simulink model "HANcoder_E407_GTSync_v4"  (R2018b)
settings: Solver=FixedStepDiscrete  StartTime=0.0  StopTime=1  FixedStep=0.01  RelTol=1e-3
PreLoadFcn:
  | librarySetup
  | eval([bdroot,'_startup']) %Calling [modelName]_startup.m
values from neighbouring files (symbols this model uses):
  basic_cycle_duration = TM12 + COMP_duration    (= 495)    [HANcoder_E407_GTSync_v4_startup.m]
  COM_Period = 100    [HANcoder_E407_GTSync_v4_startup.m]
  COM_Phase = COM_Period/2    (= 50)    [HANcoder_E407_GTSync_v4_startup.m]
  comm_delay_estimation = 20    [HANcoder_E407_GTSync_v4_startup.m]
  frequency_IRQ = 20    [HANcoder_E407_GTSync_v4_startup.m]
  HANtuneOverride = Simulink.Parameter    [HANcoder_E407_GTSync_v4_startup.m]
  idle_time_init = basic_cycle_duration*matrix_rows    (= 990)    [HANcoder_E407_GTSync_v4_startup.m]
  LED_ticks_toggle = 10000    [HANcoder_E407_GTSync_v4_startup.m]
  Master_Role = 1    [HANcoder_E407_GTSync_v4_startup.m]
  matrix_rows = 2    [HANcoder_E407_GTSync_v4_startup.m]
  Slave_Role = 2    [HANcoder_E407_GTSync_v4_startup.m]
  Sync_ID = 1    [HANcoder_E407_GTSync_v4_startup.m]
  time_difference_threshold = 500    [HANcoder_E407_GTSync_v4_startup.m]
  TM0 = basic_cycle_start    (= 5)    [HANcoder_E407_GTSync_v4_startup.m]
  TM1 = TM0 + COMM_duration    (= 105)    [HANcoder_E407_GTSync_v4_startup.m]
  TM10 = TM9  + COMP_duration    (= 465)    [HANcoder_E407_GTSync_v4_startup.m]
  TM11 = TM10 + COMP_duration    (= 475)    [HANcoder_E407_GTSync_v4_startup.m]
  TM12 = TM11 + COMP_duration    (= 485)    [HANcoder_E407_GTSync_v4_startup.m]
  TM2 = TM1 + COMP_duration    (= 115)    [HANcoder_E407_GTSync_v4_startup.m]
  TM3 = TM2 + COMP_duration    (= 125)    [HANcoder_E407_GTSync_v4_startup.m]
  TM4 = TM3 + COMM_duration    (= 225)    [HANcoder_E407_GTSync_v4_startup.m]
  TM5 = TM4 + COMP_duration    (= 235)    [HANcoder_E407_GTSync_v4_startup.m]
  TM6 = TM5 + COMM_duration    (= 335)    [HANcoder_E407_GTSync_v4_startup.m]
  TM7 = TM6 + COMP_duration    (= 345)    [HANcoder_E407_GTSync_v4_startup.m]
  TM8 = TM7 + COMM_duration    (= 445)    [HANcoder_E407_GTSync_v4_startup.m]
  TM9 = TM8  + COMP_duration    (= 455)    [HANcoder_E407_GTSync_v4_startup.m]
  Vote1_ID = 12    [HANcoder_E407_GTSync_v4_startup.m]
  Vote2_ID = 22    [HANcoder_E407_GTSync_v4_startup.m]
  Vote3_ID = 32    [HANcoder_E407_GTSync_v4_startup.m]
  wrap_up_threshold = basic_cycle_duration - time_difference_threshold*10    (= -4505)    [HANcoder_E407_GTSync_v4_startup.m]
undefined symbols (not defined in the file or in its folder): A0, A1, CON2
libraries: HANcoder_STM32_Target x22, simulink x3, hdlsllib x2, simulink_extras x1
(part 2 of 5)

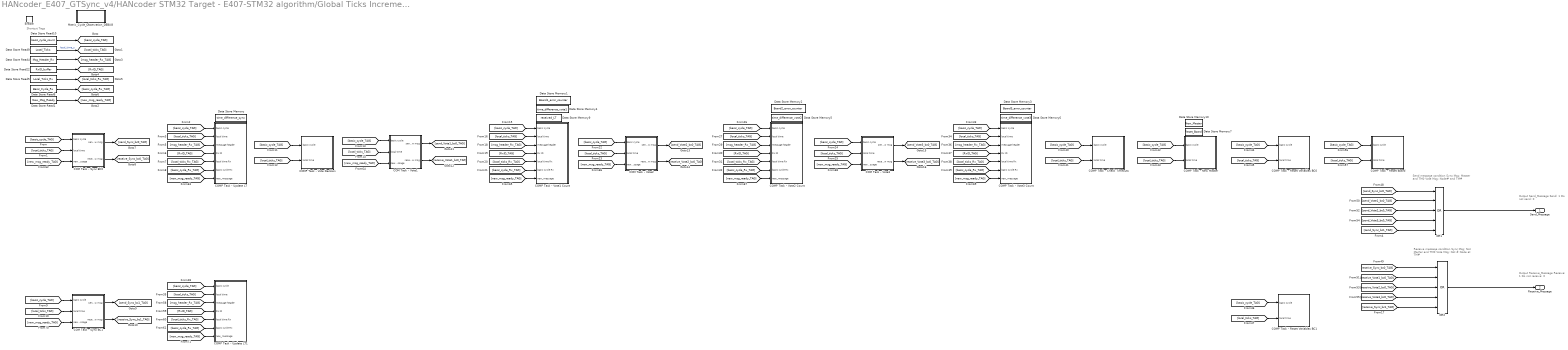
== system HANcoder_E407_GTSync_v4/HANcoder STM32 Target - E407-STM32 algorithm/Global Ticks Increment/CAN Management/Matrix Cycle Manager ==
  note: Receive message condition
      | Sync Msg: Not Master and TM0
      | Vote Msg: Not # Node at TM#
  note: Shortcut Tags
  note: Output Send_Message
      | Send: 1
      | Do not send: 0
  note: Send message condition
      | Sync Msg: Master and TM0
      | Vote Msg: Node# and TM#
  note: Output Receive_Message
      | Receive: 1
      | Do not receive: 0
  Enable : EnablePort  PropagateVarSize=During execution
  COM Task - Sync BC0 : Subsystem
  COM Task - Sync BC1 : Subsystem
  COM Task - Vote1 : Subsystem
  COM Task - Vote2 : Subsystem
  COM Task - Vote3 : Subsystem
  COMP Task - Check Timeouts : Subsystem
  COMP Task - New Master : Subsystem
  COMP Task - Reset Board : Subsystem
  COMP Task - Reset Variables BC0 : Subsystem
  COMP Task - Reset Variables BC1 : Subsystem
  COMP Task - Update LT : Subsystem
  COMP Task - Update LT1 : Subsystem
  COMP Task - Vote Decision : Subsystem
  COMP Task - Vote1 Count : Subsystem
  COMP Task - Vote2 Count : Subsystem
  COMP Task - Vote3 Count : Subsystem
  Data Store Memory : DataStoreMemory  DataStoreName=time_difference_sync  ReadBeforeWriteMsg=warning  WriteAfterWriteMsg=warning  WriteAfterReadMsg=warning  ShowAdditionalParam=off
  Data Store Memory1 : DataStoreMemory  DataStoreName=Board1_error_counter  ReadBeforeWriteMsg=warning  WriteAfterWriteMsg=warning  WriteAfterReadMsg=warning  ShowAdditionalParam=off  OutMin=0  OutMax=4294967294  OutDataTypeStr=double
  Data Store Memory10 : DataStoreMemory  DataStoreName=New_Master  ReadBeforeWriteMsg=warning  WriteAfterWriteMsg=warning  WriteAfterReadMsg=warning  ShowAdditionalParam=off  OutDataTypeStr=boolean
  Data Store Memory2 : DataStoreMemory  DataStoreName=Board2_error_counter  ReadBeforeWriteMsg=warning  WriteAfterWriteMsg=warning  WriteAfterReadMsg=warning  ShowAdditionalParam=off  OutMin=0  OutMax=4294967294  OutDataTypeStr=double
  Data Store Memory3 : DataStoreMemory  DataStoreName=Board3_error_counter  ReadBeforeWriteMsg=warning  WriteAfterWriteMsg=warning  WriteAfterReadMsg=warning  ShowAdditionalParam=off  OutMin=0  OutMax=4294967294  OutDataTypeStr=double
  Data Store Memory4 : DataStoreMemory  DataStoreName=time_difference_vote1  ReadBeforeWriteMsg=warning  WriteAfterWriteMsg=warning  WriteAfterReadMsg=warning  ShowAdditionalParam=off
  Data Store Memory5 : DataStoreMemory  DataStoreName=time_difference_vote2  ReadBeforeWriteMsg=warning  WriteAfterWriteMsg=warning  WriteAfterReadMsg=warning  ShowAdditionalParam=off
  Data Store Memory6 : DataStoreMemory  DataStoreName=time_difference_vote3  ReadBeforeWriteMsg=warning  WriteAfterWriteMsg=warning  WriteAfterReadMsg=warning  ShowAdditionalParam=off
  Data Store Memory7 : DataStoreMemory  DataStoreName=Reset_Board  ReadBeforeWriteMsg=warning  WriteAfterWriteMsg=warning  WriteAfterReadMsg=warning  ShowAdditionalParam=off  OutDataTypeStr=boolean
  Data Store Memory9 : DataStoreMemory  DataStoreName=received_LT  ReadBeforeWriteMsg=warning  WriteAfterWriteMsg=warning  WriteAfterReadMsg=warning  ShowAdditionalParam=off  OutDataTypeStr=Bus: received_vote_local_time
  Data Store Read1 : DataStoreRead  DataStoreName=New_Msg_Ready
  Data Store Read10 : DataStoreRead  DataStoreName=basic_cycle_count
  Data Store Read22 : DataStoreRead  DataStoreName=RxID_buffer
  Data Store Read4 : DataStoreRead  DataStoreName=Msg_Header_Rx
  Data Store Read5 : DataStoreRead  DataStoreName=Local_Ticks_Rx
  Data Store Read6 : DataStoreRead  DataStoreName=Basic_Cycle_Rx
  Data Store Read9 : DataStoreRead  DataStoreName=Local_Ticks
  Matrix_Cycle_Observation_DEBUG : Subsystem
  OR1 : Logic  Operator=OR  Inputs=5  IconShape=distinctive  AllPortsSameDT=off  OutDataTypeStr=boolean
  OR2 : Logic  Operator=OR  Inputs=5  IconShape=distinctive  AllPortsSameDT=off  OutDataTypeStr=boolean
  Send_Message : Outport
  Receive_Message : Outport  Port=2
  wires:
  Data Store Read10/1 -> [basic_cycle_TAG]
  OR1/1 -> Send_Message/1
  Data Store Read9/1 -> [local_ticks_TAG]  "local_time_s"
  Data Store Read4/1 -> [msg_header_Rx_TAG]
  Data Store Read22/1 -> [RxID_TAG]
  Data Store Read5/1 -> [local_ticks_Rx_TAG]
  Data Store Read6/1 -> [basic_cycle_Rx_TAG]
  [basic_cycle_TAG] -> COM Task - Sync BC0/1(basic cycle)
  [local_ticks_TAG] -> COM Task - Sync BC0/2(local time)
  [basic_cycle_TAG] -> COMP Task - Update LT/1(basic cycle)
  [local_ticks_TAG] -> COMP Task - Update LT/2(local time)
  COM Task - Sync BC0/1(send new msg) -> [send_Sync_bc0_TAG]
  COM Task - Sync BC0/2(receive new msg) -> [receive_Sync_bc0_TAG]
  [msg_header_Rx_TAG] -> COMP Task - Update LT/3(message header)
  [RxID_TAG] -> COMP Task - Update LT/4(Rx ID)
  [local_ticks_Rx_TAG] -> COMP Task - Update LT/5(local time Rx)
  [basic_cycle_Rx_TAG] -> COMP Task - Update LT/6(basic cycle Rx)
  COM Task - Sync BC1/2(receive new msg) -> [receive_Sync_bc1_TAG]
  COM Task - Sync BC1/1(send new msg) -> [send_Sync_bc1_TAG]
  [local_ticks_TAG] -> COM Task - Sync BC1/2(local time)
  [basic_cycle_TAG] -> COM Task - Sync BC1/1(basic cycle)
  [local_ticks_TAG] -> COMP Task - Vote Decision/2(local time)
  [basic_cycle_TAG] -> COMP Task - Vote Decision/1(basic cycle)
  COM Task - Vote1/2(receive new msg) -> [receive_Vote1_bc0_TAG]
  COM Task - Vote1/1(send new msg) -> [send_Vote1_bc0_TAG]
  [local_ticks_TAG] -> COM Task - Vote1/2(local time)
  [basic_cycle_TAG] -> COM Task - Vote1/1(basic cycle)
  [basic_cycle_Rx_TAG] -> COMP Task - Vote1 Count/6(basic cycle Rx)
  [local_ticks_Rx_TAG] -> COMP Task - Vote1 Count/5(local time Rx)
  [RxID_TAG] -> COMP Task - Vote1 Count/4(Rx ID)
  [msg_header_Rx_TAG] -> COMP Task - Vote1 Count/3(message header)
  [local_ticks_TAG] -> COMP Task - Vote1 Count/2(local time)
  [basic_cycle_TAG] -> COMP Task - Vote1 Count/1(basic cycle)
  [basic_cycle_TAG] -> COM Task - Vote2/1(basic cycle)
  [local_ticks_TAG] -> COM Task - Vote2/2(local time)
  COM Task - Vote2/1(send new msg) -> [send_Vote2_bc0_TAG]
  COM Task - Vote2/2(receive new msg) -> [receive_Vote2_bc0_TAG]
  COM Task - Vote3/2(receive new msg) -> [receive_Vote3_bc0_TAG]
  COM Task - Vote3/1(send new msg) -> [send_Vote3_bc0_TAG]
  [local_ticks_TAG] -> COM Task - Vote3/2(local time)
  [basic_cycle_TAG] -> COM Task - Vote3/1(basic cycle)
  [basic_cycle_TAG] -> COMP Task - Vote2 Count/1(basic cycle)
  [local_ticks_TAG] -> COMP Task - Vote2 Count/2(local time)
  [msg_header_Rx_TAG] -> COMP Task - Vote2 Count/3(message header)
  [RxID_TAG] -> COMP Task - Vote2 Count/4(Rx ID)
  [local_ticks_Rx_TAG] -> COMP Task - Vote2 Count/5(local time Rx)
  [basic_cycle_Rx_TAG] -> COMP Task - Vote2 Count/6(basic cycle Rx)
  [basic_cycle_Rx_TAG] -> COMP Task - Vote3 Count/6(basic cycle Rx)
  [local_ticks_Rx_TAG] -> COMP Task - Vote3 Count/5(local time Rx)
  [RxID_TAG] -> COMP Task - Vote3 Count/4(Rx ID)
  [msg_header_Rx_TAG] -> COMP Task - Vote3 Count/3(message header)
  [local_ticks_TAG] -> COMP Task - Vote3 Count/2(local time)
  [basic_cycle_TAG] -> COMP Task - Vote3 Count/1(basic cycle)
  [basic_cycle_TAG] -> COMP Task - Check Timeouts/1(basic cycle)
  [local_ticks_TAG] -> COMP Task - Check Timeouts/2(local time)
  [local_ticks_TAG] -> COMP Task - New Master/2(local time)
  [basic_cycle_TAG] -> COMP Task - New Master/1(basic cycle)
  [basic_cycle_TAG] -> COMP Task - Reset Variables BC0/1(basic cycle)
  [local_ticks_TAG] -> COMP Task - Reset Variables BC0/2(local time)
  [local_ticks_TAG] -> COMP Task - Reset Variables BC1/2(local time)
  [basic_cycle_TAG] -> COMP Task - Reset Variables BC1/1(basic cycle)
  [send_Sync_bc0_TAG] -> OR1/1
  [send_Vote1_bc0_TAG] -> OR1/2
  [send_Vote2_bc0_TAG] -> OR1/3
  [send_Vote3_bc0_TAG] -> OR1/4
  [receive_Vote3_bc0_TAG] -> OR2/4
  [receive_Vote2_bc0_TAG] -> OR2/3
  [receive_Vote1_bc0_TAG] -> OR2/2
  [receive_Sync_bc0_TAG] -> OR2/1
  [local_ticks_TAG] -> COMP Task - Reset Board/2(local time)
  [basic_cycle_TAG] -> COMP Task - Reset Board/1(basic cycle)
  OR2/1 -> Receive_Message/1
  [send_Sync_bc1_TAG] -> OR1/5
  [receive_Sync_bc1_TAG] -> OR2/5
  [basic_cycle_Rx_TAG] -> COMP Task - Update LT1/6(basic cycle Rx)
  [local_ticks_Rx_TAG] -> COMP Task - Update LT1/5(local time Rx)
  [RxID_TAG] -> COMP Task - Update LT1/4(Rx ID)
  [msg_header_Rx_TAG] -> COMP Task - Update LT1/3(message header)
  [local_ticks_TAG] -> COMP Task - Update LT1/2(local time)
  [basic_cycle_TAG] -> COMP Task - Update LT1/1(basic cycle)
  Data Store Read1/1 -> [new_msg_ready_TAG]
  [new_msg_ready_TAG] -> COM Task - Sync BC0/3(new_message)
  [new_msg_ready_TAG] -> COMP Task - Update LT/7(new_message)
  [new_msg_ready_TAG] -> COM Task - Vote1/3(new_message)
  [new_msg_ready_TAG] -> COMP Task - Vote1 Count/7(new_message)
  [new_msg_ready_TAG] -> COM Task - Vote2/3(new_message)
  [new_msg_ready_TAG] -> COMP Task - Vote2 Count/7(new_message)
  [new_msg_ready_TAG] -> COM Task - Vote3/3(new_message)
  [new_msg_ready_TAG] -> COMP Task - Vote3 Count/7(new_message)
  [new_msg_ready_TAG] -> COM Task - Sync BC1/3(new_message)
  [new_msg_ready_TAG] -> COMP Task - Update LT1/7(new_message)

== system HANcoder_E407_GTSync_v4/HANcoder STM32 Target - E407-STM32 algorithm/Global Ticks Increment/CAN Recieve/Buffer ready ==
  note: CAN_Rx - Buffer
      | ready for new message
  note: Logic Analyzer - DEBUG
      | Rx Buffer Ready
  Enable : EnablePort
  Data Store Write : DataStoreWrite  DataStoreName=Rx_State
  Data Store Write1 : DataStoreWrite  DataStoreName=Toggle_Pin
  New_Msg : Constant  Value=2  OutDataTypeStr=uint8
  SET : Constant  OutDataTypeStr=boolean
  wires:
  New_Msg/1 -> Data Store Write/1
  SET/1 -> Data Store Write1/1

== system HANcoder_E407_GTSync_v4/HANcoder STM32 Target - E407-STM32 algorithm/Global Ticks Increment/CAN Recieve/Prepare buffer ==
  note: Start preparing the buffer
  note: Logic Analyzer - DEBUG
      | Preparing Rx buffer
  Enable : EnablePort
  Constant1 : Constant  OutDataTypeStr=uint8
  Data Store Write : DataStoreWrite  DataStoreName=Rx_State
  Data Store Write1 : DataStoreWrite  DataStoreName=Toggle_Pin
  SET : Constant  OutDataTypeStr=boolean
  wires:
  Constant1/1 -> Data Store Write/1
  SET/1 -> Data Store Write1/1

== system HANcoder_E407_GTSync_v4/HANcoder STM32 Target - E407-STM32 algorithm/Global Ticks Increment/CAN Recieve/RxID_CAN ==
  RxID : Inport
  Bus Creator4 : BusCreator  Inputs=8
  Bus Selector : BusSelector  OutputSignals=signal1,signal2,signal3,signal4,signal5,signal6,signal7,signal8,signal9
  Bus Creator{,1..3} (4 alike) : BusCreator  Inputs=9
  Constant : Constant  Value=Sync_ID
  Constant1 : Constant  Value=Vote1_ID
  Constant2 : Constant  Value=Vote2_ID
  Constant3 : Constant  Value=Vote3_ID
  Equal{,1..3} (4 alike) : RelationalOperator  Operator===  OutDataTypeStr=boolean  RndMeth=Simplest
  Switch : Switch  Criteria=u2 > Threshold
  Switch1 : Switch  Criteria=u2 > Threshold
  Switch2 : Switch  Criteria=u2 > Threshold
  Sync_ID_CAN : Subsystem
  Vote1_ID_CAN : Subsystem
  Vote2_ID_CAN : Subsystem
  Vote3_ID_CAN : Subsystem
  CAN_new : Outport
  message : Outport  Port=2
  wires:
  Constant/1 -> Equal/2
  RxID/1 -> Equal2/1, Equal3/1, Equal1/1, Equal/1
  Equal/1 -> Sync_ID_CAN/Enable, Switch/2
  Constant1/1 -> Equal1/2
  Constant2/1 -> Equal2/2
  Constant3/1 -> Equal3/2
  Equal1/1 -> Vote1_ID_CAN/Enable, Switch1/2
  Equal2/1 -> Vote2_ID_CAN/Enable, Switch2/2
  Equal3/1 -> Vote3_ID_CAN/Enable
  Sync_ID_CAN/1(CAN_new) -> Bus Creator/1
  Sync_ID_CAN/2(Out2) -> Bus Creator/2
  Sync_ID_CAN/3(Out3) -> Bus Creator/3
  Sync_ID_CAN/4(Out4) -> Bus Creator/4
  Sync_ID_CAN/5(Out5) -> Bus Creator/5
  Sync_ID_CAN/6(Out6) -> Bus Creator/6
  Sync_ID_CAN/7(Out7) -> Bus Creator/7
  Sync_ID_CAN/8(Out8) -> Bus Creator/8
  Sync_ID_CAN/9(Out9) -> Bus Creator/9
  Bus Creator/1 -> Switch/1
  Vote1_ID_CAN/1(CAN_new) -> Bus Creator1/1
  Vote1_ID_CAN/2(Out2) -> Bus Creator1/2
  Vote1_ID_CAN/3(Out3) -> Bus Creator1/3
  Vote1_ID_CAN/4(Out4) -> Bus Creator1/4
  Vote1_ID_CAN/5(Out5) -> Bus Creator1/5
  Vote1_ID_CAN/6(Out6) -> Bus Creator1/6
  Vote1_ID_CAN/7(Out7) -> Bus Creator1/7
  Vote1_ID_CAN/8(Out8) -> Bus Creator1/8
  Vote1_ID_CAN/9(Out9) -> Bus Creator1/9
  Bus Creator1/1 -> Switch1/1
  Vote2_ID_CAN/1(CAN_new) -> Bus Creator2/1
  Vote2_ID_CAN/2(Out2) -> Bus Creator2/2
  Vote2_ID_CAN/3(Out3) -> Bus Creator2/3
  Vote2_ID_CAN/4(Out4) -> Bus Creator2/4
  Vote2_ID_CAN/6(Out6) -> Bus Creator2/6
  Vote2_ID_CAN/5(Out5) -> Bus Creator2/5
  Vote2_ID_CAN/7(Out7) -> Bus Creator2/7
  Vote2_ID_CAN/8(Out8) -> Bus Creator2/8
  Vote2_ID_CAN/9(Out9) -> Bus Creator2/9
  Bus Creator2/1 -> Switch2/1
  Vote3_ID_CAN/1(CAN_new) -> Bus Creator3/1
  Vote3_ID_CAN/2(Out2) -> Bus Creator3/2
  Vote3_ID_CAN/3(Out3) -> Bus Creator3/3
  Vote3_ID_CAN/4(Out4) -> Bus Creator3/4
  Vote3_ID_CAN/5(Out5) -> Bus Creator3/5
  Vote3_ID_CAN/6(Out6) -> Bus Creator3/6
  Vote3_ID_CAN/7(Out7) -> Bus Creator3/7
  Vote3_ID_CAN/8(Out8) -> Bus Creator3/8
  Vote3_ID_CAN/9(Out9) -> Bus Creator3/9
  Bus Creator3/1 -> Switch2/3
  Switch1/1 -> Switch/3
  Switch2/1 -> Switch1/3
  Switch/1 -> Bus Selector/1
  Bus Selector/1 -> CAN_new/1  "<signal1>"
  Bus Creator4/1 -> message/1
  Bus Selector/2 -> Bus Creator4/1  "<signal2>"
  Bus Selector/3 -> Bus Creator4/2  "<signal3>"
  Bus Selector/4 -> Bus Creator4/3  "<signal4>"
  Bus Selector/5 -> Bus Creator4/4  "<signal5>"
  Bus Selector/6 -> Bus Creator4/5  "<signal6>"
  Bus Selector/7 -> Bus Creator4/6  "<signal7>"
  Bus Selector/8 -> Bus Creator4/7  "<signal8>"
  Bus Selector/9 -> Bus Creator4/8  "<signal9>"

== system HANcoder_E407_GTSync_v4/HANcoder STM32 Target - E407-STM32 algorithm/Global Ticks Increment/CAN Recieve/Update message buffers ==
  note: Local time when the
      | message is received
  note: Received message
      | ready for processing
  note: CAN_Rx stop listening
  note: Logic Analyzer - DEBUG
      | Message received!
  message : Inport
  Enable : EnablePort
  Data Store Write : DataStoreWrite  DataStoreName=Toggle_Pin
  Data Store Write1 : DataStoreWrite  DataStoreName=Msg_Header_Rx
  Data Store Write2 : DataStoreWrite  DataStoreName=New_Msg_Ready
  Data Store Write3 : DataStoreWrite  DataStoreName=Local_Ticks_Rx
  Data Store Write4 : DataStoreWrite  DataStoreName=Basic_Cycle_Rx
  Data Store Write5 : DataStoreWrite  DataStoreName=Rx_State
  Data Store Write6 : DataStoreWrite  DataStoreName=Msg_Rx_Ticks
  Data Type Conversion{1..9} (9 alike) : DataTypeConversion  OutDataTypeStr=double
  Demux : Demux  Outputs=8
  Idle_State : Constant  Value=3  OutDataTypeStr=uint8
  Local_Time : DataStoreRead  DataStoreName=Local_Ticks
  SET : Constant  OutDataTypeStr=boolean
  Terminator{1..8} (8 alike) : Terminator
  UINT8 to UINT16 : Subsystem
  wires:
  UINT8 to UINT16/1(Out1) -> Data Type Conversion2/1, Data Store Write3/1  "received_local_time_update"
  Demux/4 -> Data Store Write4/1, Data Type Conversion5/1
  Idle_State/1 -> Data Store Write5/1
  Demux/8 -> Data Type Conversion9/1
  Demux/7 -> Data Type Conversion8/1
  Demux/3 -> UINT8 to UINT16/2(In2), Data Type Conversion4/1
  Data Type Conversion7/1 -> Terminator3/1  "received_message_2"
  Demux/1 -> Data Type Conversion3/1
  Data Type Conversion9/1 -> Terminator7/1  "received_message_4"
  Demux/5 -> Data Type Conversion6/1
  Demux/6 -> Data Type Conversion7/1
  Data Type Conversion5/1 -> Terminator1/1  "received_basic_cycle"
  Demux/2 -> UINT8 to UINT16/1(In1), Data Type Conversion1/1
  Data Type Conversion1/1 -> Terminator8/1  "received_local_time_1"
  Data Type Conversion2/1 -> Terminator5/1  "received_local_time"
  Data Type Conversion3/1 -> Data Store Write1/1  "Message_Header_s"
  Data Type Conversion8/1 -> Terminator6/1  "received_message_3"
  Data Type Conversion6/1 -> Terminator4/1  "received_message_1"
  Data Type Conversion4/1 -> Terminator2/1  "received_local_time_2"
  message/1 -> Demux/1
  SET/1 -> Data Store Write/1, Data Store Write2/1
  Local_Time/1 -> Data Store Write6/1

== system HANcoder_E407_GTSync_v4/HANcoder STM32 Target - E407-STM32 algorithm/Global Ticks Increment/CAN Send/CAN send ==
  In1 : Inport
  In2 : Inport  Port=2
  In3 : Inport  Port=3
  In4 : Inport  Port=4
  In5 : Inport  Port=5
  In6 : Inport  Port=6
  In7 : Inport  Port=7
  In8 : Inport  Port=8
  In9 : Inport  Port=9
  S-Function : M-S-Function  FunctionName=sfcn_can_send  Parameters=tsamp, canBus, frameType, inputNumber, dataType, byteOrder
  wires:
  In1/1 -> S-Function/1
  In2/1 -> S-Function/2
  In3/1 -> S-Function/3
  In4/1 -> S-Function/4
  In5/1 -> S-Function/5
  In6/1 -> S-Function/6
  In7/1 -> S-Function/7
  In8/1 -> S-Function/8
  In9/1 -> S-Function/9

== system HANcoder_E407_GTSync_v4/HANcoder STM32 Target - E407-STM32 algorithm/Global Ticks Increment/CAN Send/UINT16 to UINT8 ==
  In1 : Inport
  Bit Shift : hdlsllib/Logic and Bit Operations/Bit Shift  mode=Shift Right Logical  N=8
      settings: SourceProductName=HDL Coder  SourceProductBaseCode=HD
  Cast6 : DataTypeConversion  OutDataTypeStr=uint8
  Cast7 : DataTypeConversion  OutDataTypeStr=uint8
  Out1 : Outport
  Out2 : Outport  Port=2
  wires:
  In1/1 -> Bit Shift/1, Cast7/1
  Bit Shift/1 -> Cast6/1
  Cast6/1 -> Out2/1
  Cast7/1 -> Out1/1

== system HANcoder_E407_GTSync_v4/HANcoder STM32 Target - E407-STM32 algorithm/Global Ticks Increment/CAN Management/Initialization/Delay ==
  note: Update counter
      | < +1 tick every activation >
  note: Reset local counter
      | < for next activation >
  note: End of Delay
  Input : Inport
  Add2 : Sum
  Data Store Read : DataStoreRead  DataStoreName=Delay_Counter
  Data Store Read1 : DataStoreRead  DataStoreName=Delay_Counter
  Data Store Write2 : DataStoreWrite  DataStoreName=Delay_Counter
  GreaterThan : RelationalOperator  OutDataTypeStr=boolean  RndMeth=Simplest
  Increment1 : Constant  OutDataTypeStr=double
  Initializaton_Observation_DEBUG : Subsystem
  Reset : Constant  Value=-1  OutDataTypeStr=double
  Switch : Switch  Criteria=u2 > Threshold
  Output : Outport
  wires:
  Data Store Read/1 -> Add2/1
  Increment1/1 -> Add2/2
  Data Store Read1/1 -> GreaterThan/1
  Input/1 -> GreaterThan/2
  GreaterThan/1 -> Switch/2, Output/1
  Add2/1 -> Switch/3
  Reset/1 -> Switch/1
  Switch/1 -> Data Store Write2/1

== system HANcoder_E407_GTSync_v4/HANcoder STM32 Target - E407-STM32 algorithm/Global Ticks Increment/CAN Management/Initialization/RoleID and Global Time init ==
  note: Sync msg received!
  note: Reset variables
  note: Finish Initialization
  note: Role_ID Initialization
  Timeout Initialization : Inport
  Reference message received : Inport  Port=2
  Enable : EnablePort
  Constant : Constant  Value=Master_Role
  Constant1 : Constant  Value=Slave_Role
  Data Store Read : DataStoreRead  DataStoreName=Role_ID
  Data Store Write : DataStoreWrite  DataStoreName=Role_ID
  Data Store Write1 : DataStoreWrite  DataStoreName=sync_processed
  Data Store Write2 : DataStoreWrite  DataStoreName=Delay_Counter
  Data Store Write3 : DataStoreWrite  DataStoreName=New_Msg_Ready
  Data Store Write4 : DataStoreWrite  DataStoreName=Initialization_Timeout
  Global Time Initialization Master : Subsystem
  Global Time Initialization Slave : Subsystem
  RESET : Constant  Value=0  OutDataTypeStr=boolean
  RESET1 : Constant  Value=0  OutDataTypeStr=double
  RESET2 : Constant  Value=0  OutDataTypeStr=boolean
  SET : Constant
  SET1 : Constant  OutDataTypeStr=boolean
  Switch1 : Switch  Criteria=u2 > Threshold
  Switch2 : Switch  Criteria=u2 > Threshold
  Finish Initialization : Outport  OutputWhenDisabled=reset  InitialOutput=0
  wires:
  Switch1/1 -> Switch2/3
  Reference message received/1 -> Switch2/2, Global Time Initialization Slave/Enable
  Data Store Read/1 -> Switch1/3
  SET/1 -> Finish Initialization/1
  Constant/1 -> Switch1/1
  Constant1/1 -> Switch2/1
  Switch2/1 -> Data Store Write/1
  RESET/1 -> Data Store Write4/1
  Timeout Initialization/1 -> Global Time Initialization Master/Enable, Switch1/2
  RESET1/1 -> Data Store Write2/1
  SET1/1 -> Data Store Write1/1
  RESET2/1 -> Data Store Write3/1

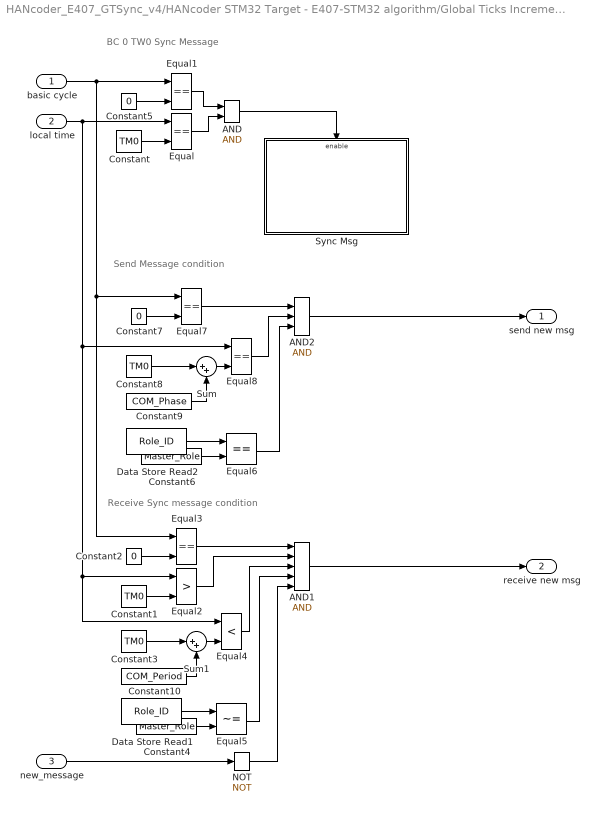
== system HANcoder_E407_GTSync_v4/HANcoder STM32 Target - E407-STM32 algorithm/Global Ticks Increment/CAN Management/Matrix Cycle Manager/COM Task - Sync BC0 ==
  note: BC 0 TW0
      | Sync Message
  note: Receive Sync message condition
  note: Send Message condition
  basic cycle : Inport
  local time : Inport  Port=2
  new_message : Inport  Port=3
  AND : Logic  IconShape=distinctive  AllPortsSameDT=off  OutDataTypeStr=boolean
  AND1 : Logic  Inputs=5  IconShape=distinctive  AllPortsSameDT=off  OutDataTypeStr=boolean
  AND2 : Logic  Inputs=3  IconShape=distinctive  AllPortsSameDT=off  OutDataTypeStr=boolean
  Constant{,1,3,8} (4 alike) : Constant  Value=TM0
  Constant10 : Constant  Value=COM_Period
  Constant2 : Constant  Value=0  OutDataTypeStr=uint8
  Constant4 : Constant  Value=Master_Role
  Constant5 : Constant  Value=0
  Constant6 : Constant  Value=Master_Role
  Constant7 : Constant  Value=0
  Constant9 : Constant  Value=COM_Phase
  Data Store Read1 : DataStoreRead  DataStoreName=Role_ID
  Data Store Read2 : DataStoreRead  DataStoreName=Role_ID
  Equal{,1,3,6..8} (6 alike) : RelationalOperator  Operator===  OutDataTypeStr=boolean  RndMeth=Simplest
  Equal2 : RelationalOperator  Operator=>  OutDataTypeStr=boolean  RndMeth=Simplest
  Equal4 : RelationalOperator  Operator=<  OutDataTypeStr=boolean  RndMeth=Simplest
  Equal5 : RelationalOperator  Operator=~=  OutDataTypeStr=boolean  RndMeth=Simplest
  NOT : Logic  Operator=NOT  IconShape=distinctive  AllPortsSameDT=off  OutDataTypeStr=boolean
  Sum : Sum  Inputs=|++
  Sum1 : Sum  Inputs=|++
  Sync Msg : Subsystem
  send new msg : Outport
  receive new msg : Outport  Port=2
  wires:
  Constant/1 -> Equal/2
  Constant5/1 -> Equal1/2
  Equal1/1 -> AND/1
  Equal/1 -> AND/2
  AND/1 -> Sync Msg/Enable
  Data Store Read1/1 -> Equal5/1
  Constant4/1 -> Equal5/2
  basic cycle/1 -> Equal7/1, Equal3/1, Equal1/1
  AND1/1 -> receive new msg/1
  local time/1 -> Equal4/1, Equal2/1, Equal8/1, Equal/1
  Equal2/1 -> AND1/2
  Equal5/1 -> AND1/4
  Equal3/1 -> AND1/1
  Equal4/1 -> AND1/3
  Constant3/1 -> Sum1/1
  Constant1/1 -> Equal2/2
  Constant2/1 -> Equal3/2
  Constant6/1 -> Equal6/2
  Data Store Read2/1 -> Equal6/1
  Constant7/1 -> Equal7/2
  Equal7/1 -> AND2/1
  AND2/1 -> send new msg/1
  Equal8/1 -> AND2/2
  Equal6/1 -> AND2/3
  Constant8/1 -> Sum/1
  Sum/1 -> Equal8/2
  Constant9/1 -> Sum/2
  Constant10/1 -> Sum1/2
  Sum1/1 -> Equal4/2
  new_message/1 -> NOT/1
  NOT/1 -> AND1/5

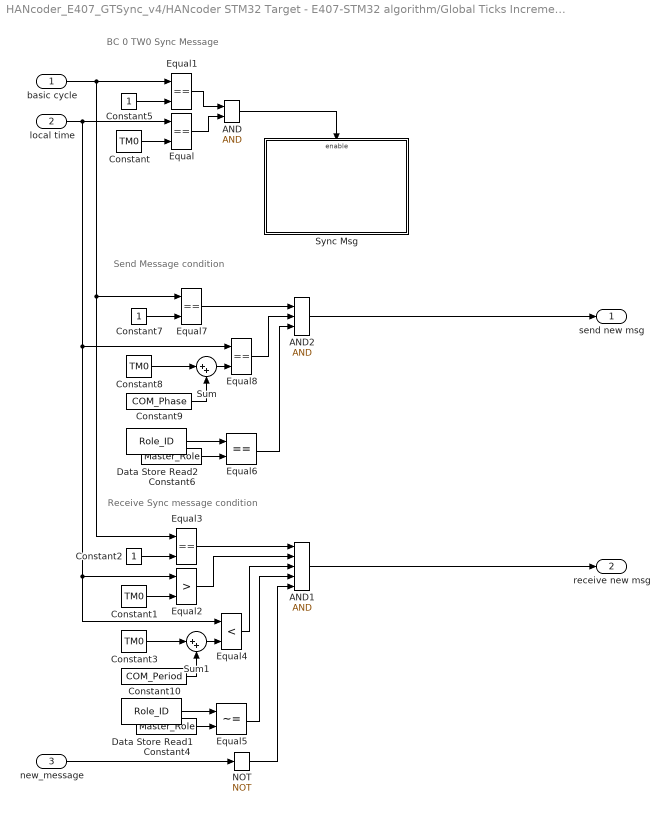
== system HANcoder_E407_GTSync_v4/HANcoder STM32 Target - E407-STM32 algorithm/Global Ticks Increment/CAN Management/Matrix Cycle Manager/COM Task - Sync BC1 ==
  note: BC 0 TW0
      | Sync Message
  note: Receive Sync message condition
  note: Send Message condition
  basic cycle : Inport
  local time : Inport  Port=2
  new_message : Inport  Port=3
  AND : Logic  IconShape=distinctive  AllPortsSameDT=off  OutDataTypeStr=boolean
  AND1 : Logic  Inputs=5  IconShape=distinctive  AllPortsSameDT=off  OutDataTypeStr=boolean
  AND2 : Logic  Inputs=3  IconShape=distinctive  AllPortsSameDT=off  OutDataTypeStr=boolean
  Constant{,1,3,8} (4 alike) : Constant  Value=TM0
  Constant10 : Constant  Value=COM_Period
  Constant2 : Constant  OutDataTypeStr=uint8
  Constant4 : Constant  Value=Master_Role
  Constant5 : Constant
  Constant6 : Constant  Value=Master_Role
  Constant7 : Constant
  Constant9 : Constant  Value=COM_Phase
  Data Store Read1 : DataStoreRead  DataStoreName=Role_ID
  Data Store Read2 : DataStoreRead  DataStoreName=Role_ID
  Equal{,1,3,6..8} (6 alike) : RelationalOperator  Operator===  OutDataTypeStr=boolean  RndMeth=Simplest
  Equal2 : RelationalOperator  Operator=>  OutDataTypeStr=boolean  RndMeth=Simplest
  Equal4 : RelationalOperator  Operator=<  OutDataTypeStr=boolean  RndMeth=Simplest
  Equal5 : RelationalOperator  Operator=~=  OutDataTypeStr=boolean  RndMeth=Simplest
  NOT : Logic  Operator=NOT  IconShape=distinctive  AllPortsSameDT=off  OutDataTypeStr=boolean
  Sum : Sum  Inputs=|++
  Sum1 : Sum  Inputs=|++
  Sync Msg : Subsystem
  send new msg : Outport
  receive new msg : Outport  Port=2
  wires:
  Constant/1 -> Equal/2
  Constant5/1 -> Equal1/2
  Equal1/1 -> AND/1
  Equal/1 -> AND/2
  AND/1 -> Sync Msg/Enable
  Data Store Read1/1 -> Equal5/1
  Constant4/1 -> Equal5/2
  basic cycle/1 -> Equal7/1, Equal3/1, Equal1/1
  local time/1 -> Equal4/1, Equal2/1, Equal8/1, Equal/1
  Equal2/1 -> AND1/2
  Equal5/1 -> AND1/4
  Equal3/1 -> AND1/1
  Equal4/1 -> AND1/3
  Constant3/1 -> Sum1/1
  Constant1/1 -> Equal2/2
  Constant2/1 -> Equal3/2
  Constant6/1 -> Equal6/2
  Data Store Read2/1 -> Equal6/1
  Constant7/1 -> Equal7/2
  Equal7/1 -> AND2/1
  Equal8/1 -> AND2/2
  Equal6/1 -> AND2/3
  Constant8/1 -> Sum/1
  Sum/1 -> Equal8/2
  Constant9/1 -> Sum/2
  Constant10/1 -> Sum1/2
  Sum1/1 -> Equal4/2
  new_message/1 -> NOT/1
  NOT/1 -> AND1/5
  AND1/1 -> receive new msg/1
  AND2/1 -> send new msg/1

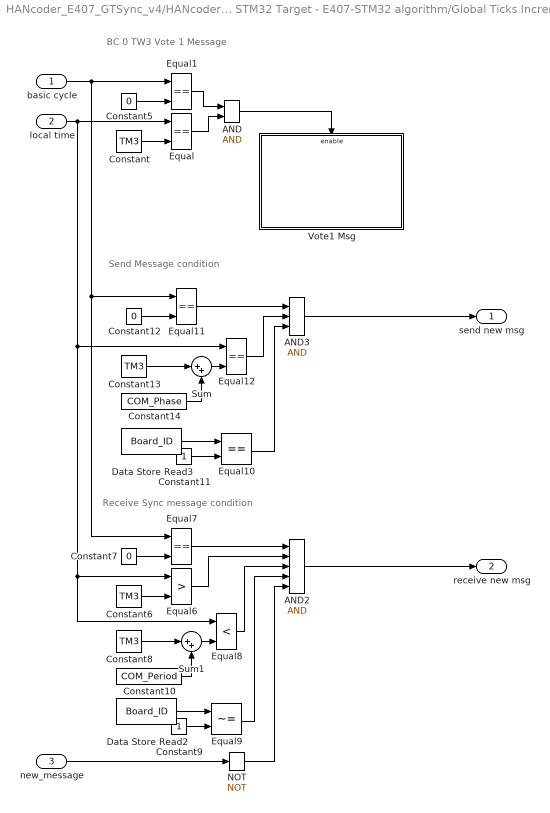
== system HANcoder_E407_GTSync_v4/HANcoder STM32 Target - E407-STM32 algorithm/Global Ticks Increment/CAN Management/Matrix Cycle Manager/COM Task - Vote1 ==
  note: BC 0 TW3
      | Vote 1 Message
  note: Send Message condition
  note: Receive Sync message condition
  basic cycle : Inport
  local time : Inport  Port=2
  new_message : Inport  Port=3
  AND : Logic  IconShape=distinctive  AllPortsSameDT=off  OutDataTypeStr=boolean
  AND2 : Logic  Inputs=5  IconShape=distinctive  AllPortsSameDT=off  OutDataTypeStr=boolean
  AND3 : Logic  Inputs=3  IconShape=distinctive  AllPortsSameDT=off  OutDataTypeStr=boolean
  Constant{,6,8,13} (4 alike) : Constant  Value=TM3
  Constant10 : Constant  Value=COM_Period
  Constant11 : Constant
  Constant12 : Constant  Value=0
  Constant14 : Constant  Value=COM_Phase
  Constant5 : Constant  Value=0
  Constant7 : Constant  Value=0  OutDataTypeStr=uint8
  Constant9 : Constant
  Data Store Read2 : DataStoreRead  DataStoreName=Board_ID
  Data Store Read3 : DataStoreRead  DataStoreName=Board_ID
  Equal{,1,7,10..12} (6 alike) : RelationalOperator  Operator===  OutDataTypeStr=boolean  RndMeth=Simplest
  Equal6 : RelationalOperator  Operator=>  OutDataTypeStr=boolean  RndMeth=Simplest
  Equal8 : RelationalOperator  Operator=<  OutDataTypeStr=boolean  RndMeth=Simplest
  Equal9 : RelationalOperator  Operator=~=  OutDataTypeStr=boolean  RndMeth=Simplest
  NOT : Logic  Operator=NOT  IconShape=distinctive  AllPortsSameDT=off  OutDataTypeStr=boolean
  Sum : Sum  Inputs=|++
  Sum1 : Sum  Inputs=|++
  Vote1 Msg : Subsystem
  send new msg : Outport
  receive new msg : Outport  Port=2
  wires:
  AND/1 -> Vote1 Msg/Enable
  Equal/1 -> AND/2
  Equal1/1 -> AND/1
  Constant5/1 -> Equal1/2
  Constant/1 -> Equal/2
  Constant11/1 -> Equal10/2
  Sum/1 -> Equal12/2
  Constant13/1 -> Sum/1
  Constant6/1 -> Equal6/2
  Constant7/1 -> Equal7/2
  Constant9/1 -> Equal9/2
  Equal9/1 -> AND2/4
  basic cycle/1 -> Equal11/1, Equal7/1, Equal1/1
  local time/1 -> Equal/1, Equal12/1, Equal8/1, Equal6/1
  Data Store Read2/1 -> Equal9/1
  Equal8/1 -> AND2/3
  Equal7/1 -> AND2/1
  Equal6/1 -> AND2/2
  Equal12/1 -> AND3/2
  Data Store Read3/1 -> Equal10/1
  Constant10/1 -> Sum1/2
  Constant8/1 -> Sum1/1
  Equal10/1 -> AND3/3
  Sum1/1 -> Equal8/2
  Constant12/1 -> Equal11/2
  Constant14/1 -> Sum/2
  Equal11/1 -> AND3/1
  new_message/1 -> NOT/1
  NOT/1 -> AND2/5
  AND3/1 -> send new msg/1
  AND2/1 -> receive new msg/1

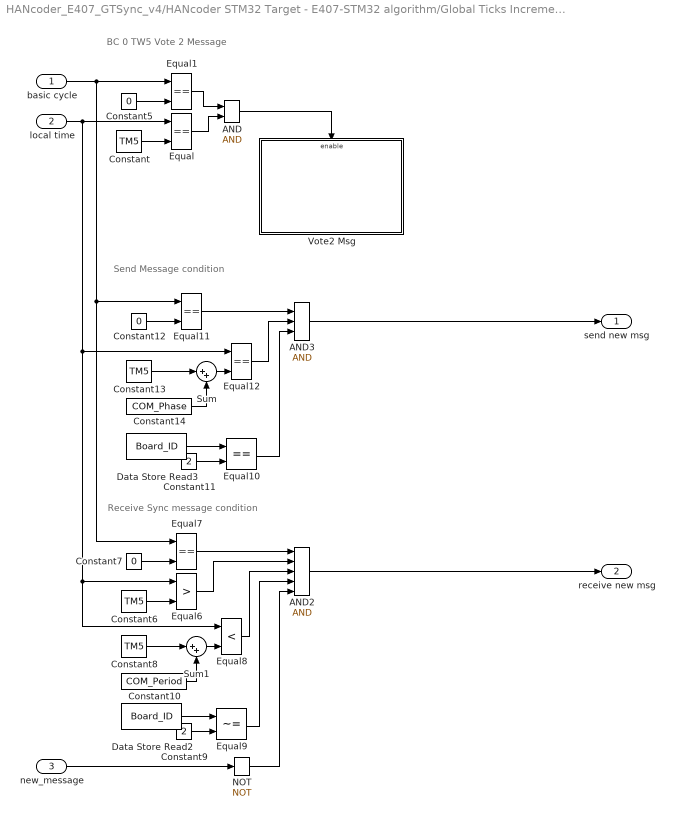
== system HANcoder_E407_GTSync_v4/HANcoder STM32 Target - E407-STM32 algorithm/Global Ticks Increment/CAN Management/Matrix Cycle Manager/COM Task - Vote2 ==
  note: BC 0 TW5
      | Vote 2 Message
  note: Receive Sync message condition
  note: Send Message condition
  basic cycle : Inport
  local time : Inport  Port=2
  new_message : Inport  Port=3
  AND : Logic  IconShape=distinctive  AllPortsSameDT=off  OutDataTypeStr=boolean
  AND2 : Logic  Inputs=5  IconShape=distinctive  AllPortsSameDT=off  OutDataTypeStr=boolean
  AND3 : Logic  Inputs=3  IconShape=distinctive  AllPortsSameDT=off  OutDataTypeStr=boolean
  Constant{,6,8,13} (4 alike) : Constant  Value=TM5
  Constant10 : Constant  Value=COM_Period
  Constant11 : Constant  Value=2
  Constant12 : Constant  Value=0
  Constant14 : Constant  Value=COM_Phase
  Constant5 : Constant  Value=0
  Constant7 : Constant  Value=0  OutDataTypeStr=uint8
  Constant9 : Constant  Value=2
  Data Store Read2 : DataStoreRead  DataStoreName=Board_ID
  Data Store Read3 : DataStoreRead  DataStoreName=Board_ID
  Equal{,1,7,10..12} (6 alike) : RelationalOperator  Operator===  OutDataTypeStr=boolean  RndMeth=Simplest
  Equal6 : RelationalOperator  Operator=>  OutDataTypeStr=boolean  RndMeth=Simplest
  Equal8 : RelationalOperator  Operator=<  OutDataTypeStr=boolean  RndMeth=Simplest
  Equal9 : RelationalOperator  Operator=~=  OutDataTypeStr=boolean  RndMeth=Simplest
  NOT : Logic  Operator=NOT  IconShape=distinctive  AllPortsSameDT=off  OutDataTypeStr=boolean
  Sum : Sum  Inputs=|++
  Sum1 : Sum  Inputs=|++
  Vote2 Msg : Subsystem
  send new msg : Outport
  receive new msg : Outport  Port=2
  wires:
  Constant/1 -> Equal/2
  Constant5/1 -> Equal1/2
  Equal1/1 -> AND/1
  Equal/1 -> AND/2
  AND/1 -> Vote2 Msg/Enable
  basic cycle/1 -> Equal11/1, Equal7/1, Equal1/1
  Constant12/1 -> Equal11/2
  Equal11/1 -> AND3/1
  Constant14/1 -> Sum/2
  Constant10/1 -> Sum1/2
  Equal10/1 -> AND3/3
  Sum1/1 -> Equal8/2
  Constant8/1 -> Sum1/1
  Data Store Read3/1 -> Equal10/1
  Equal12/1 -> AND3/2
  Equal6/1 -> AND2/2
  Equal8/1 -> AND2/3
  Data Store Read2/1 -> Equal9/1
  Equal9/1 -> AND2/4
  Constant7/1 -> Equal7/2
  Equal7/1 -> AND2/1
  Constant13/1 -> Sum/1
  Constant11/1 -> Equal10/2
  Sum/1 -> Equal12/2
  local time/1 -> Equal12/1, Equal8/1, Equal6/1, Equal/1
  Constant6/1 -> Equal6/2
  Constant9/1 -> Equal9/2
  new_message/1 -> NOT/1
  NOT/1 -> AND2/5
  AND3/1 -> send new msg/1
  AND2/1 -> receive new msg/1

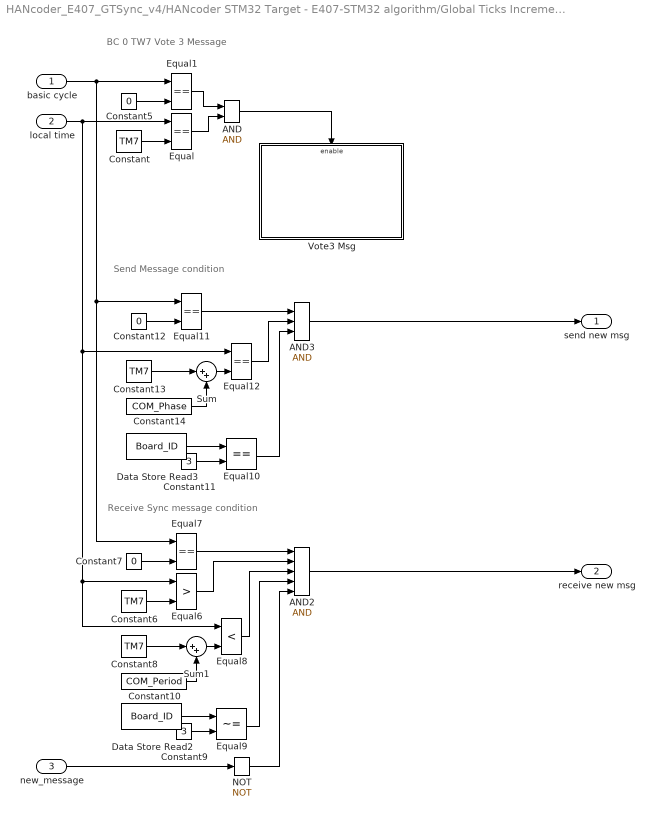
== system HANcoder_E407_GTSync_v4/HANcoder STM32 Target - E407-STM32 algorithm/Global Ticks Increment/CAN Management/Matrix Cycle Manager/COM Task - Vote3 ==
  note: BC 0 TW7
      | Vote 3 Message
  note: Receive Sync message condition
  note: Send Message condition
  basic cycle : Inport
  local time : Inport  Port=2
  new_message : Inport  Port=3
  AND : Logic  IconShape=distinctive  AllPortsSameDT=off  OutDataTypeStr=boolean
  AND2 : Logic  Inputs=5  IconShape=distinctive  AllPortsSameDT=off  OutDataTypeStr=boolean
  AND3 : Logic  Inputs=3  IconShape=distinctive  AllPortsSameDT=off  OutDataTypeStr=boolean
  Constant{,6,8,13} (4 alike) : Constant  Value=TM7
  Constant10 : Constant  Value=COM_Period
  Constant11 : Constant  Value=3
  Constant12 : Constant  Value=0
  Constant14 : Constant  Value=COM_Phase
  Constant5 : Constant  Value=0
  Constant7 : Constant  Value=0  OutDataTypeStr=uint8
  Constant9 : Constant  Value=3
  Data Store Read2 : DataStoreRead  DataStoreName=Board_ID
  Data Store Read3 : DataStoreRead  DataStoreName=Board_ID
  Equal{,1,7,10..12} (6 alike) : RelationalOperator  Operator===  OutDataTypeStr=boolean  RndMeth=Simplest
  Equal6 : RelationalOperator  Operator=>  OutDataTypeStr=boolean  RndMeth=Simplest
  Equal8 : RelationalOperator  Operator=<  OutDataTypeStr=boolean  RndMeth=Simplest
  Equal9 : RelationalOperator  Operator=~=  OutDataTypeStr=boolean  RndMeth=Simplest
  NOT : Logic  Operator=NOT  IconShape=distinctive  AllPortsSameDT=off  OutDataTypeStr=boolean
  Sum : Sum  Inputs=|++
  Sum1 : Sum  Inputs=|++
  Vote3 Msg : Subsystem
  send new msg : Outport
  receive new msg : Outport  Port=2
  wires:
  AND/1 -> Vote3 Msg/Enable
  Equal/1 -> AND/2
  Equal1/1 -> AND/1
  Constant5/1 -> Equal1/2
  Constant/1 -> Equal/2
  AND2/1 -> receive new msg/1
  basic cycle/1 -> Equal11/1, Equal7/1, Equal1/1
  Constant12/1 -> Equal11/2
  Equal11/1 -> AND3/1
  Constant14/1 -> Sum/2
  Constant10/1 -> Sum1/2
  Equal10/1 -> AND3/3
  Sum1/1 -> Equal8/2
  Constant8/1 -> Sum1/1
  Data Store Read3/1 -> Equal10/1
  Equal12/1 -> AND3/2
  Equal6/1 -> AND2/2
  Equal8/1 -> AND2/3
  Data Store Read2/1 -> Equal9/1
  Equal9/1 -> AND2/4
  Constant7/1 -> Equal7/2
  Equal7/1 -> AND2/1
  Constant13/1 -> Sum/1
  Constant11/1 -> Equal10/2
  Sum/1 -> Equal12/2
  local time/1 -> Equal12/1, Equal8/1, Equal6/1, Equal/1
  Constant6/1 -> Equal6/2
  Constant9/1 -> Equal9/2
  new_message/1 -> NOT/1
  NOT/1 -> AND2/5
  AND3/1 -> send new msg/1

== system HANcoder_E407_GTSync_v4/HANcoder STM32 Target - E407-STM32 algorithm/Global Ticks Increment/CAN Management/Matrix Cycle Manager/COMP Task - Check Timeouts ==
  note: BC 0 TW9
      | Timeout check
  basic cycle : Inport
  local time : Inport  Port=2
  AND : Logic  IconShape=distinctive  AllPortsSameDT=off  OutDataTypeStr=boolean
  Constant : Constant  Value=TM9
  Constant5 : Constant  Value=0
  Equal : RelationalOperator  Operator===  OutDataTypeStr=boolean  RndMeth=Simplest
  Equal1 : RelationalOperator  Operator===  OutDataTypeStr=boolean  RndMeth=Simplest
  Timeout and Board error counter : Subsystem
  wires:
  Constant/1 -> Equal/2
  local time/1 -> Equal/1
  Constant5/1 -> Equal1/2
  basic cycle/1 -> Equal1/1
  Equal1/1 -> AND/1
  Equal/1 -> AND/2
  AND/1 -> Timeout and Board error counter/Enable

== system HANcoder_E407_GTSync_v4/HANcoder STM32 Target - E407-STM32 algorithm/Global Ticks Increment/CAN Management/Matrix Cycle Manager/COMP Task - New Master ==
  note: BC 0 TW10
      | New Master decision
  basic cycle : Inport
  local time : Inport  Port=2
  AND : Logic  IconShape=distinctive  AllPortsSameDT=off  OutDataTypeStr=boolean
  Constant : Constant  Value=TM10
  Constant5 : Constant  Value=0
  Equal : RelationalOperator  Operator===  OutDataTypeStr=boolean  RndMeth=Simplest
  Equal1 : RelationalOperator  Operator===  OutDataTypeStr=boolean  RndMeth=Simplest
  New Master : Subsystem
  wires:
  AND/1 -> New Master/Enable
  Equal/1 -> AND/2
  Equal1/1 -> AND/1
  basic cycle/1 -> Equal1/1
  Constant5/1 -> Equal1/2
  local time/1 -> Equal/1
  Constant/1 -> Equal/2

== system HANcoder_E407_GTSync_v4/HANcoder STM32 Target - E407-STM32 algorithm/Global Ticks Increment/CAN Management/Matrix Cycle Manager/COMP Task - Reset Board ==
  note: BC 0 TW12
      | Reset Board
  basic cycle : Inport
  local time : Inport  Port=2
  AND : Logic  Inputs=3  IconShape=distinctive  AllPortsSameDT=off  OutDataTypeStr=boolean
  Constant : Constant  Value=TM12
  Constant5 : Constant  Value=0
  Data Store Read : DataStoreRead  DataStoreName=Reset_Board
  Equal : RelationalOperator  Operator===  OutDataTypeStr=boolean  RndMeth=Simplest
  Equal1 : RelationalOperator  Operator===  OutDataTypeStr=boolean  RndMeth=Simplest
  RESET Board - Return to initialization : Subsystem  TreatAsAtomicUnit=on
  wires:
  AND/1 -> RESET Board - Return to initialization/Enable
  Equal/1 -> AND/2
  Equal1/1 -> AND/1
  basic cycle/1 -> Equal1/1
  Constant5/1 -> Equal1/2
  local time/1 -> Equal/1
  Constant/1 -> Equal/2
  Data Store Read/1 -> AND/3

== system HANcoder_E407_GTSync_v4/HANcoder STM32 Target - E407-STM32 algorithm/Global Ticks Increment/CAN Management/Matrix Cycle Manager/COMP Task - Reset Variables BC0 ==
  note: BC 0 TW11
      | Reset variables
  basic cycle : Inport
  local time : Inport  Port=2
  AND : Logic  IconShape=distinctive  AllPortsSameDT=off  OutDataTypeStr=boolean
  Constant : Constant  Value=TM11
  Constant5 : Constant  Value=0
  Equal : RelationalOperator  Operator===  OutDataTypeStr=boolean  RndMeth=Simplest
  Equal1 : RelationalOperator  Operator===  OutDataTypeStr=boolean  RndMeth=Simplest
  Reset variables : Subsystem
  wires:
  Constant/1 -> Equal/2
  local time/1 -> Equal/1
  Constant5/1 -> Equal1/2
  basic cycle/1 -> Equal1/1
  Equal1/1 -> AND/1
  Equal/1 -> AND/2
  AND/1 -> Reset variables/Enable

== system HANcoder_E407_GTSync_v4/HANcoder STM32 Target - E407-STM32 algorithm/Global Ticks Increment/CAN Management/Matrix Cycle Manager/COMP Task - Reset Variables BC1 ==
  note: BC 1 TW11
      | Reset Variables
  basic cycle : Inport
  local time : Inport  Port=2
  AND : Logic  IconShape=distinctive  AllPortsSameDT=off  OutDataTypeStr=boolean
  Constant : Constant  Value=TM11
  Constant5 : Constant
  Equal : RelationalOperator  Operator===  OutDataTypeStr=boolean  RndMeth=Simplest
  Equal1 : RelationalOperator  Operator===  OutDataTypeStr=boolean  RndMeth=Simplest
  Reset Variables : Subsystem
  wires:
  AND/1 -> Reset Variables/Enable
  Equal/1 -> AND/2
  Equal1/1 -> AND/1
  basic cycle/1 -> Equal1/1
  Constant5/1 -> Equal1/2
  local time/1 -> Equal/1
  Constant/1 -> Equal/2

== system HANcoder_E407_GTSync_v4/HANcoder STM32 Target - E407-STM32 algorithm/Global Ticks Increment/CAN Management/Matrix Cycle Manager/COMP Task - Update LT ==
  note: Sync Message
      | received by Slave
  note: BC 0 TW1
      | Sync Message
  basic cycle : Inport
  local time : Inport  Port=2
  message header : Inport  Port=3
  Rx ID : Inport  Port=4
  local time Rx : Inport  Port=5
  basic cycle Rx : Inport  Port=6
  new_message : Inport  Port=7
  AND : Logic  IconShape=distinctive  AllPortsSameDT=off  OutDataTypeStr=boolean
  AND1 : Logic  IconShape=distinctive  AllPortsSameDT=off  OutDataTypeStr=boolean
  AND12 : Logic  Inputs=3  IconShape=distinctive  AllPortsSameDT=off  OutDataTypeStr=boolean
  Constant : Constant  Value=TM1
  Constant4 : Constant  Value=Slave_Role
  Constant5 : Constant  Value=0
  Data Store Memory : DataStoreMemory  DataStoreName=LT_Update_Counter  ReadBeforeWriteMsg=warning  WriteAfterWriteMsg=warning  WriteAfterReadMsg=warning  ShowAdditionalParam=off
  Data Store Read1 : DataStoreRead  DataStoreName=Role_ID
  Equal{,1..2,18} (4 alike) : RelationalOperator  Operator===  OutDataTypeStr=boolean  RndMeth=Simplest
  Local Time Update : Subsystem
  SyncID1 : Constant  Value=Sync_ID
  Terminator : Terminator
  wires:
  Constant4/1 -> Equal2/2
  Data Store Read1/1 -> Equal2/1
  AND12/1 -> AND1/2
  local time Rx/1 -> Local Time Update/1(Local Time Rx)
  Rx ID/1 -> Equal18/1
  basic cycle Rx/1 -> Local Time Update/2(Basic_Cycle_Rx)
  Equal18/1 -> AND12/2
  SyncID1/1 -> Equal18/2
  Equal2/1 -> AND12/3
  message header/1 -> Terminator/1
  Equal1/1 -> AND/1
  basic cycle/1 -> Equal1/1
  Constant/1 -> Equal/2
  local time/1 -> Equal/1
  Equal/1 -> AND/2
  Constant5/1 -> Equal1/2
  AND1/1 -> Local Time Update/Enable
  AND/1 -> AND1/1
  new_message/1 -> AND12/1

== system HANcoder_E407_GTSync_v4/HANcoder STM32 Target - E407-STM32 algorithm/Global Ticks Increment/CAN Management/Matrix Cycle Manager/COMP Task - Update LT1 ==
  note: BC 1 TW1
      | Sync Message
  note: Sync Message
      | received by Slave
  basic cycle : Inport
  local time : Inport  Port=2
  message header : Inport  Port=3
  Rx ID : Inport  Port=4
  local time Rx : Inport  Port=5
  basic cycle Rx : Inport  Port=6
  new_message : Inport  Port=7
  AND : Logic  IconShape=distinctive  AllPortsSameDT=off  OutDataTypeStr=boolean
  AND1 : Logic  IconShape=distinctive  AllPortsSameDT=off  OutDataTypeStr=boolean
  AND12 : Logic  Inputs=3  IconShape=distinctive  AllPortsSameDT=off  OutDataTypeStr=boolean
  Constant : Constant  Value=TM1
  Constant4 : Constant  Value=Slave_Role
  Constant5 : Constant
  Data Store Read1 : DataStoreRead  DataStoreName=Role_ID
  Equal{,1..2,18} (4 alike) : RelationalOperator  Operator===  OutDataTypeStr=boolean  RndMeth=Simplest
  Local Time Update : Subsystem
  SyncID1 : Constant  Value=Sync_ID
  Terminator : Terminator
  wires:
  AND/1 -> AND1/1
  AND1/1 -> Local Time Update/Enable
  Constant5/1 -> Equal1/2
  Equal/1 -> AND/2
  local time/1 -> Equal/1
  Constant/1 -> Equal/2
  basic cycle/1 -> Equal1/1
  Equal1/1 -> AND/1
  message header/1 -> Terminator/1
  Equal2/1 -> AND12/3
  SyncID1/1 -> Equal18/2
  Equal18/1 -> AND12/2
  basic cycle Rx/1 -> Local Time Update/2(Basic_Cycle_Rx)
  Rx ID/1 -> Equal18/1
  local time Rx/1 -> Local Time Update/1(Local Time Rx)
  AND12/1 -> AND1/2
  Data Store Read1/1 -> Equal2/1
  Constant4/1 -> Equal2/2
  new_message/1 -> AND12/1

== system HANcoder_E407_GTSync_v4/HANcoder STM32 Target - E407-STM32 algorithm/Global Ticks Increment/CAN Management/Matrix Cycle Manager/COMP Task - Vote Decision ==
  note: BC 0 TW2
      | Vote decision
  basic cycle : Inport
  local time : Inport  Port=2
  AND : Logic  IconShape=distinctive  AllPortsSameDT=off  OutDataTypeStr=boolean
  Constant : Constant  Value=TM2
  Constant5 : Constant  Value=0
  Equal : RelationalOperator  Operator===  OutDataTypeStr=boolean  RndMeth=Simplest
  Equal1 : RelationalOperator  Operator===  OutDataTypeStr=boolean  RndMeth=Simplest
  Vote Decision : Subsystem
  wires:
  AND/1 -> Vote Decision/Enable
  Equal/1 -> AND/2
  Equal1/1 -> AND/1
  basic cycle/1 -> Equal1/1
  Constant5/1 -> Equal1/2
  local time/1 -> Equal/1
  Constant/1 -> Equal/2

== system HANcoder_E407_GTSync_v4/HANcoder STM32 Target - E407-STM32 algorithm/Global Ticks Increment/CAN Management/Matrix Cycle Manager/COMP Task - Vote1 Count ==
  note: BC 0 TW4
      | Vote 1 Message
  note: Vote 1 received by
      | other boards
  basic cycle : Inport
  local time : Inport  Port=2
  message header : Inport  Port=3
  Rx ID : Inport  Port=4
  local time Rx : Inport  Port=5
  basic cycle Rx : Inport  Port=6
  new_message : Inport  Port=7
  AND : Logic  IconShape=distinctive  AllPortsSameDT=off  OutDataTypeStr=boolean
  AND1 : Logic  IconShape=distinctive  AllPortsSameDT=off  OutDataTypeStr=boolean
  AND12 : Logic  Inputs=3  IconShape=distinctive  AllPortsSameDT=off  OutDataTypeStr=boolean
  Constant : Constant  Value=TM4
  Constant4 : Constant
  Constant5 : Constant  Value=0
  Data Store Read1 : DataStoreRead  DataStoreName=Board_ID
  Equal : RelationalOperator  Operator===  OutDataTypeStr=boolean  RndMeth=Simplest
  Equal1 : RelationalOperator  Operator===  OutDataTypeStr=boolean  RndMeth=Simplest
  Equal18 : RelationalOperator  Operator===  OutDataTypeStr=boolean  RndMeth=Simplest
  Equal2 : RelationalOperator  Operator=~=  OutDataTypeStr=boolean  RndMeth=Simplest
  RxID : Constant  Value=Vote1_ID
  Terminator : Terminator
  Vote Count 1 : Subsystem
  wires:
  AND/1 -> AND1/1
  AND1/1 -> Vote Count 1/Enable
  Constant5/1 -> Equal1/2
  Equal/1 -> AND/2
  local time/1 -> Equal/1
  Constant/1 -> Equal/2
  basic cycle/1 -> Equal1/1
  Equal1/1 -> AND/1
  message header/1 -> Vote Count 1/1(Msg Header)
  Equal2/1 -> AND12/3
  RxID/1 -> Equal18/2
  Equal18/1 -> AND12/2
  Rx ID/1 -> Equal18/1
  local time Rx/1 -> Vote Count 1/2(Local Time Rx)
  AND12/1 -> AND1/2
  Data Store Read1/1 -> Equal2/1
  Constant4/1 -> Equal2/2
  basic cycle Rx/1 -> Terminator/1
  new_message/1 -> AND12/1

== system HANcoder_E407_GTSync_v4/HANcoder STM32 Target - E407-STM32 algorithm/Global Ticks Increment/CAN Management/Matrix Cycle Manager/COMP Task - Vote2 Count ==
  note: Vote 2 received by
      | other boards
  note: BC 0 TW6
      | Vote 1 Message
  basic cycle : Inport
  local time : Inport  Port=2
  message header : Inport  Port=3
  Rx ID : Inport  Port=4
  local time Rx : Inport  Port=5
  basic cycle Rx : Inport  Port=6
  new_message : Inport  Port=7
  AND : Logic  IconShape=distinctive  AllPortsSameDT=off  OutDataTypeStr=boolean
  AND1 : Logic  IconShape=distinctive  AllPortsSameDT=off  OutDataTypeStr=boolean
  AND12 : Logic  Inputs=3  IconShape=distinctive  AllPortsSameDT=off  OutDataTypeStr=boolean
  Constant : Constant  Value=TM6
  Constant4 : Constant  Value=2
  Constant5 : Constant  Value=0
  Data Store Read1 : DataStoreRead  DataStoreName=Board_ID
  Equal : RelationalOperator  Operator===  OutDataTypeStr=boolean  RndMeth=Simplest
  Equal1 : RelationalOperator  Operator===  OutDataTypeStr=boolean  RndMeth=Simplest
  Equal18 : RelationalOperator  Operator===  OutDataTypeStr=boolean  RndMeth=Simplest
  Equal2 : RelationalOperator  Operator=~=  OutDataTypeStr=boolean  RndMeth=Simplest
  RxID : Constant  Value=Vote2_ID
  Terminator : Terminator
  Vote Count 2 : Subsystem
  wires:
  basic cycle Rx/1 -> Terminator/1
  Constant4/1 -> Equal2/2
  Data Store Read1/1 -> Equal2/1
  AND12/1 -> AND1/2
  local time Rx/1 -> Vote Count 2/2(Local Time Rx)
  Rx ID/1 -> Equal18/1
  Equal18/1 -> AND12/2
  RxID/1 -> Equal18/2
  Equal2/1 -> AND12/3
  message header/1 -> Vote Count 2/1(Msg Header1)
  Equal1/1 -> AND/1
  basic cycle/1 -> Equal1/1
  Constant/1 -> Equal/2
  local time/1 -> Equal/1
  Equal/1 -> AND/2
  Constant5/1 -> Equal1/2
  AND1/1 -> Vote Count 2/Enable
  AND/1 -> AND1/1
  new_message/1 -> AND12/1

== system HANcoder_E407_GTSync_v4/HANcoder STM32 Target - E407-STM32 algorithm/Global Ticks Increment/CAN Management/Matrix Cycle Manager/COMP Task - Vote3 Count ==
  note: BC 0 TW8
      | Vote 3 Message
  note: Vote 3 received by
      | other boards
  basic cycle : Inport
  local time : Inport  Port=2
  message header : Inport  Port=3
  Rx ID : Inport  Port=4
  local time Rx : Inport  Port=5
  basic cycle Rx : Inport  Port=6
  new_message : Inport  Port=7
  AND : Logic  IconShape=distinctive  AllPortsSameDT=off  OutDataTypeStr=boolean
  AND1 : Logic  IconShape=distinctive  AllPortsSameDT=off  OutDataTypeStr=boolean
  AND12 : Logic  Inputs=3  IconShape=distinctive  AllPortsSameDT=off  OutDataTypeStr=boolean
  Constant : Constant  Value=TM8
  Constant4 : Constant  Value=3
  Constant5 : Constant  Value=0
  Data Store Read1 : DataStoreRead  DataStoreName=Board_ID
  Equal : RelationalOperator  Operator===  OutDataTypeStr=boolean  RndMeth=Simplest
  Equal1 : RelationalOperator  Operator===  OutDataTypeStr=boolean  RndMeth=Simplest
  Equal18 : RelationalOperator  Operator===  OutDataTypeStr=boolean  RndMeth=Simplest
  Equal2 : RelationalOperator  Operator=~=  OutDataTypeStr=boolean  RndMeth=Simplest
  RxID : Constant  Value=Vote3_ID
  Terminator : Terminator
  Vote Count 3 : Subsystem
  wires:
  AND/1 -> AND1/1
  AND1/1 -> Vote Count 3/Enable
  Constant5/1 -> Equal1/2
  Equal/1 -> AND/2
  local time/1 -> Equal/1
  Constant/1 -> Equal/2
  basic cycle/1 -> Equal1/1
  Equal1/1 -> AND/1
  message header/1 -> Vote Count 3/1(Msg Header1)
  Equal2/1 -> AND12/3
  RxID/1 -> Equal18/2
  Equal18/1 -> AND12/2
  Rx ID/1 -> Equal18/1
  local time Rx/1 -> Vote Count 3/2(Local Time Rx)
  AND12/1 -> AND1/2
  Data Store Read1/1 -> Equal2/1
  Constant4/1 -> Equal2/2
  basic cycle Rx/1 -> Terminator/1
  new_message/1 -> AND12/1
